simulink model "reto24"  (R2024a)
settings: Solver=ode4  StartTime=0.0  StopTime=10.0  FixedStep=0.003  RelTol=1e-3
settings Model: Creator=Usuario  LastModifiedBy=Usuario

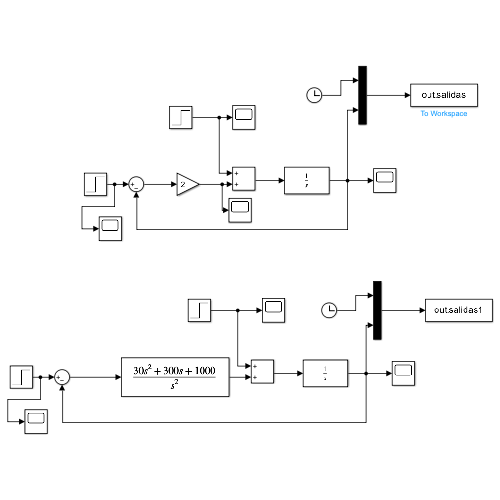
[thumbnail: Simulink's stored preview of the top-level diagram]
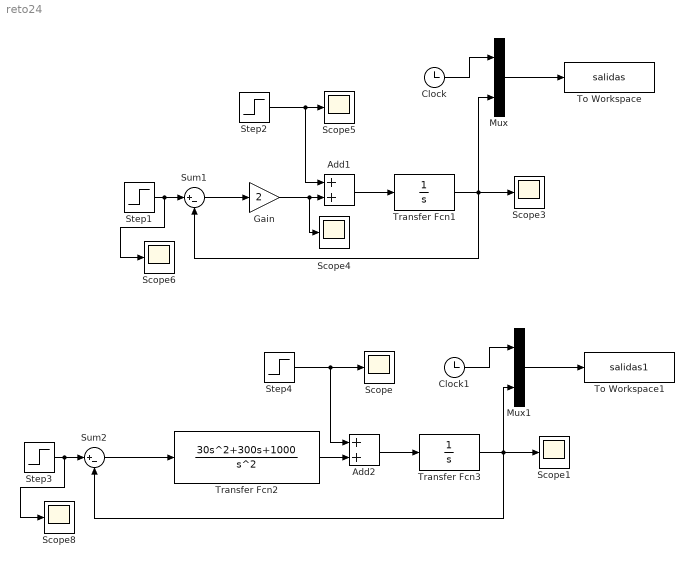
== system reto24 ==
  Add1 : Sum
  Add2 : Sum
  Clock : Clock
  Clock1 : Clock
  Gain : Gain  Gain=2
  Mux : Mux  Inputs=2
  Mux1 : Mux  Inputs=2
  Scope{,1,3..6,8} (7 alike) : Scope
  Step{1..4} (4 alike) : Step  Time=0  SampleTime=0
  Sum1 : Sum  Inputs=|+-
  Sum2 : Sum  Inputs=|+-
  To Workspace : ToWorkspace  VariableName=salidas  SampleTime=-1
  To Workspace1 : ToWorkspace  VariableName=salidas1  SampleTime=-1
  Transfer Fcn1 : TransferFcn  Denominator=[1 0]
  Transfer Fcn2 : TransferFcn  Numerator=[30 300 1000]  Denominator=[1 0 0]
  Transfer Fcn3 : TransferFcn  Denominator=[1 0]
  wires:
  Step2/1 -> Scope5/1, Add1/1
  Gain/1 -> Scope4/1, Add1/2
  Sum1/1 -> Gain/1
  Transfer Fcn1/1 -> Mux/2, Sum1/2, Scope3/1
  Mux/1 -> To Workspace/1
  Clock/1 -> Mux/1
  Add1/1 -> Transfer Fcn1/1
  Step1/1 -> Scope6/1, Sum1/1
  Step4/1 -> Scope/1, Add2/1
  Add2/1 -> Transfer Fcn3/1
  Step3/1 -> Scope8/1, Sum2/1
  Transfer Fcn3/1 -> Mux1/2, Sum2/2, Scope1/1
  Clock1/1 -> Mux1/1
  Mux1/1 -> To Workspace1/1
  Transfer Fcn2/1 -> Add2/2
  Sum2/1 -> Transfer Fcn2/1
